simulink model "CC_sfun"  (R2024b)
settings: Solver=FixedStepDiscrete  StartTime=0.0  StopTime=inf  RelTol=1e-3  EnableMultiTasking=on
undefined symbols (not defined in the file or in its folder): CCOk_stepSize
settings Model: TunableVars=CCOk_stepSize  TunableVarsStorageClass=Auto  Creator=nctzv8  LastModifiedBy=voillat
settings ConfigSet: Description=OpenECU configuration set for code generation under RTW-EC.
settings SolverCC: AlgebraicLoopSolver=TrustRegion  PositivePriorityOrder=on
settings DataIOCC: LimitDataPoints=on  SaveFormat=Array  SignalLoggingSaveFormat=ModelDataLogs
settings OptimizationCC: DefaultParameterBehavior=Inlined  InlineInvariantSignals=on  ExpressionDepthLimit=2147483647  StateBitsets=on  DataBitsets=on  ZeroExternalMemoryAtStartup=off  ZeroInternalMemoryAtStartup=off  NoFixptDivByZeroProtection=on  EfficientFloat2IntCast=on  LifeSpan=1  EfficientTunableParamExpr=on
settings DebuggingCC: SaveWithParameterizedLinksMsg=none  SignalResolutionControl=TryResolveAllWithWarning  MultiTaskDSMMsg=warning  MultiTaskCondExecSysMsg=none  SingleTaskRateTransMsg=error  CheckMatrixSingularityMsg=warning  VectorMatrixConversionMsg=warning  SignalLabelMismatchMsg=warning  UnconnectedInputMsg=warning  UnconnectedOutputMsg=warning  UnconnectedLineMsg=warning  AllowSymbolicDim=off  StateNameClashWarn=warning  SFUnexpectedBacktrackingDiag=warning  SFNoUnconditionalDefaultTransitionDiag=warning  SFExecutionAtInitializationDiag=none  ArithmeticOperatorsInVariantConditions=warning
settings HardwareCC: ProdBitPerPointer=32  ProdBitPerSizeT=32  ProdBitPerPtrDiffT=32  ProdLargestAtomicInteger=Long  ProdLargestAtomicFloat=Double  ProdEndianess=BigEndian  ProdWordSize=32  ProdHWDeviceType=Freescale->32-bit PowerPC  TargetIntDivRoundTo=Zero  TargetEndianess=BigEndian  TargetHWDeviceType=Freescale->32-bit PowerPC  ProdEqTarget=off
settings ModelReferenceCC: EnableRefExpFcnMdlSchedulingChecks=on  PropagateSignalLabelsOutOfModel=off
settings SFSimCC: SimUseLocalCustomCode=off  MATLABDynamicMemAlloc=off  CustomCodeUndefinedFunction=UseInterfaceOnly
settings RTWCC: Description=OpenECU Platform Target (ERT, optimised floating-point code)  SystemTargetFile=openecu_ert.tlc  MakeCommand=make_rtw optimized_floating_point=1  TemplateMakefile=openecu_ert_r2015b_64.tmf  RetainRTWFile=on  RTWUseLocalCustomCode=off  IncludeHyperlinkInReport=on  GPUComputeCapability=3.5
settings CodeAppCC: ForceParamTrailComments=on  IgnoreCustomStorageClasses=off  SimulinkDataObjDesc=on  CustomSymbolStrType=$N$R$M  InsertBlockDesc=on  StateflowObjectComments=on  InternalIdentifier=Classic
settings STFCustomTargetCC: TargetLibSuffix=.a  GenerateSampleERTMain=on  IncludeMdlTerminateFcn=off  CombineOutputUpdateFcns=on  IncludeFileDelimiter=UseQuote  ERTCustomFileBanners=on  SupportContinuousTime=off  RemoveResetFunc=on  MATLABClassNameForMDSCustomization=Simulink.SoftwareTarget.ERTCustomization  SystemTargetFile=openecu_ert.tlc
settings ERTTargetCC: MultiwordLength=2048  GenerateSampleERTMain=on  ParMdlRefBuildCompliant=off  CompOptLevelCompliant=off  ConcurrentExecutionCompliant=off  IncludeMdlTerminateFcn=off  IncludeFileDelimiter=UseQuote  SupportNonInlinedSFcns=on  ModelStepFunctionPrototypeControlCompliant=off  CPPClassGenCompliant=off  UseToolchainInfoCompliant=off  ExtModeMexFile=noextcomm  ERTSrcFileBannerTemplate=oe_code_c_template.cgt  ERTHdrFileBannerTemplate=oe_code_h_template.cgt  ERTDataSrcFileTemplate=oe_data_c_template.cgt  ERTDataHdrFileTemplate=oe_data_h_template.cgt  ERTCustomFileTemplate=example_file_process.tlc  GlobalDataDefinition=InSeparateSourceFile  GlobalDataReference=InSeparateHeaderFile  ConvertIfToSwitch=off  SuppressUnreachableDefaultCases=off  EnableUserReplacementTypes=on  DynamicArrayContainerType=coder::array
settings ConfigComp: CovMetricSettings=dw  CovSaveCumulativeToWorkspaceVar=on  CovSaveSingleToWorkspaceVar=on  CovExternalEMLEnable=off

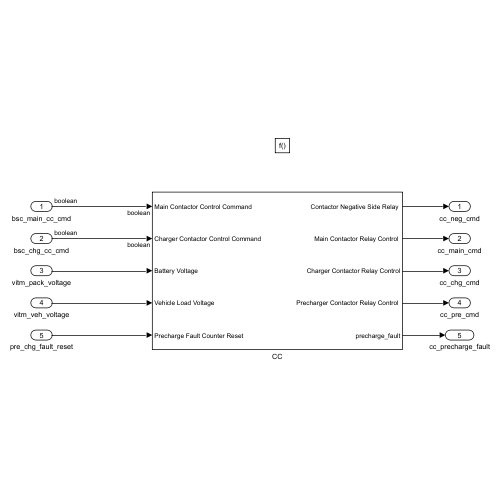
[thumbnail: Simulink's stored preview of the top-level diagram]
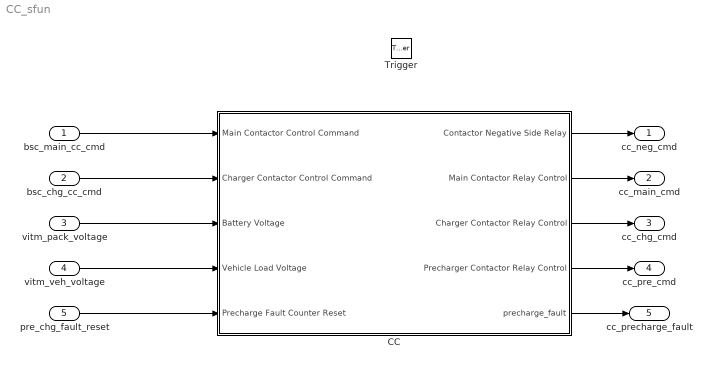
== system CC_sfun ==
  bsc_main_cc_cmd : Inport  OutDataTypeStr=boolean
  bsc_chg_cc_cmd : Inport  Port=2  OutDataTypeStr=boolean
  vitm_pack_voltage : Inport  Port=3
  vitm_veh_voltage : Inport  Port=4
  pre_chg_fault_reset : Inport  Port=5
  Trigger : TriggerPort  TriggerType=function-call  VariantControl=(inherit)  PortDimensions=1
  CC : Subsystem  mask{sfcnParam1=CCOk_stepSize}
      mask prompts: sfcnParam1 "CCOk_stepSize:"
      mask help: Simulink:masks:GenSFuncDesc_MD
      mask Help: eval('feval(''rtwprivate'',''rtwhelpview'',''rtw_sfcn_block'')');
  cc_neg_cmd : Outport
  cc_main_cmd : Outport  Port=2
  cc_chg_cmd : Outport  Port=3
  cc_pre_cmd : Outport  Port=4
  cc_precharge_fault : Outport  Port=5
  wires:
  bsc_main_cc_cmd/1 -> CC/1(Main Contactor Control Command)
  bsc_chg_cc_cmd/1 -> CC/2(Charger Contactor Control Command)
  vitm_pack_voltage/1 -> CC/3(Battery Voltage)
  vitm_veh_voltage/1 -> CC/4(Vehicle Load Voltage)
  pre_chg_fault_reset/1 -> CC/5(Precharge Fault Counter Reset)
  CC/1("Contactor Negative Side Relay ") -> cc_neg_cmd/1
  CC/2("Main Contactor Relay Control ") -> cc_main_cmd/1
  CC/3(Charger Contactor Relay Control) -> cc_chg_cmd/1
  CC/4("Precharger Contactor Relay Control ") -> cc_pre_cmd/1
  CC/5(precharge_fault) -> cc_precharge_fault/1

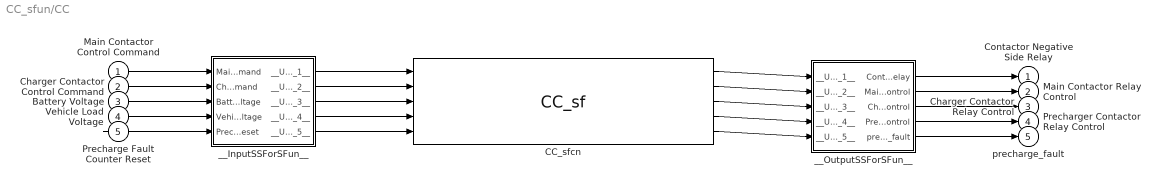
== system CC_sfun/CC ==
  Main Contactor Control Command : Inport  OutDataTypeStr=boolean
  Charger Contactor Control Command : Inport  Port=2  OutDataTypeStr=boolean
  Battery Voltage : Inport  Port=3
  Vehicle Load Voltage : Inport  Port=4
  Precharge Fault Counter Reset : Inport  Port=5
  CC_sfcn : S-Function  FunctionName=CC_sf  Parameters=sfcnParam1  SFunctionModules=""  SFunctionDeploymentMode=off  EnableBusSupport=off  mask{rtw_sf_name=CC_sf, showVar=off, sfcnParam1=sfcnParam1}
      mask prompts: rtw_sf_name "Simulink:masks:GenSFuncName_MP"; showVar "Simulink:masks:GenSFuncShowModuleList_MP"; sfcnParam1 "CCOk_stepSize:"
      mask help: Simulink:masks:GenSFuncDesc_MD
      mask init:
      | displist = '';
      | if ~strcmp(get_param(gcb, 'FunctionName'), rtw_sf_name);
      |   set_param(gcb, 'FunctionName', rtw_sf_name);
      | end
      | % Check if we are generating code
      | rtw_mode = false;
      | if strcmpi(get_param(bdroot(gcb),'SimulationStatus'),'Initializing')
      | 	rtw_mode = strcmpi(get_param(bdroot(gcb),'BuildingRTWCode'),'on') && ...
      | 		~strcmpi(get_param(bdroot(gcb),'TargetStyle'),'SimulationTarget');
      | end
      | if showVar || rtw_mode
      | 	if exist('rtwsfunc') == 2 | exist('rtwsfunc') == 6
      | 		tmplist = rtwsfunc(rtw_sf_name,gcb);
      | 		tmplist = DAStudio.message('Simulink:masks:GenSFuncListOfModules_IC', tmplist);
      | 	elseif showVar
      | 		tmplist1 = DAStudio.message('Simulink:masks:GenSFuncListOfModules_IC', '');
      |         tmplist2 = DAStudio.message('Simulink:masks:GenSFuncNotLicensed_IC');
      |         tmplist = [tmplist1 tmplist2];
      |  	end
      | end
      | if showVar
      |   displist = tmplist;
      | end
      settings: CopyFcn=|
      | if ~strcmp(get_param(gcb,'Linkstatus'),'none') && ...
      | ~strcmp(get_param(gcb,'Linkstatus'),'implicit')
      |   set_param(gcb,'LinkStatus','none');
      | end
      mask Help: eval('feval(''rtwprivate'',''rtwhelpview'',''rtw_sfcn_block'')');
      mask Display:
      | port_label('input',1,'Main Contactor Control Command');
      | port_label('input',2,'Charger Contactor Control Command');
      | port_label('input',3,'Battery Voltage');
      | port_label('input',4,'Vehicle Load Voltage');
      | port_label('input',5,'Precharge Fault Counter Reset');
      | port_label('output',1,'Contactor Negative Side Relay ');
      | port_label('output',2,'Main Contactor Relay Control ');
      | port_label('output',3,'Charger Contactor Relay Control');
      | port_label('output',4,'Precharger Contactor Relay Control ');
      | port_label('output',5,'precharge_fault');
  __InputSSForSFun__ : Subsystem
  __OutputSSForSFun__ : Subsystem
  "Contactor Negative Side Relay " : Outport
  "Main Contactor Relay Control " : Outport  Port=2
  Charger Contactor Relay Control : Outport  Port=3
  "Precharger Contactor Relay Control " : Outport  Port=4
  precharge_fault : Outport  Port=5
  wires:
  Main Contactor Control Command/1 -> __InputSSForSFun__/1(Main Contactor Control Command)
  Charger Contactor Control Command/1 -> __InputSSForSFun__/2(Charger Contactor Control Command)
  Battery Voltage/1 -> __InputSSForSFun__/3(Battery Voltage)
  Vehicle Load Voltage/1 -> __InputSSForSFun__/4(Vehicle Load Voltage)
  Precharge Fault Counter Reset/1 -> __InputSSForSFun__/5(Precharge Fault Counter Reset)
  __InputSSForSFun__/1(__UniqueOutportName__1__) -> CC_sfcn/1
  __InputSSForSFun__/2(__UniqueOutportName__2__) -> CC_sfcn/2
  __InputSSForSFun__/3(__UniqueOutportName__3__) -> CC_sfcn/3
  __InputSSForSFun__/4(__UniqueOutportName__4__) -> CC_sfcn/4
  __InputSSForSFun__/5(__UniqueOutportName__5__) -> CC_sfcn/5
  CC_sfcn/1 -> __OutputSSForSFun__/1(__UniqueInportName__1__)
  CC_sfcn/2 -> __OutputSSForSFun__/2(__UniqueInportName__2__)
  CC_sfcn/3 -> __OutputSSForSFun__/3(__UniqueInportName__3__)
  CC_sfcn/4 -> __OutputSSForSFun__/4(__UniqueInportName__4__)
  CC_sfcn/5 -> __OutputSSForSFun__/5(__UniqueInportName__5__)
  __OutputSSForSFun__/1("Contactor Negative Side Relay ") -> "Contactor Negative Side Relay "/1
  __OutputSSForSFun__/2("Main Contactor Relay Control ") -> "Main Contactor Relay Control "/1
  __OutputSSForSFun__/3(Charger Contactor Relay Control) -> Charger Contactor Relay Control/1
  __OutputSSForSFun__/4("Precharger Contactor Relay Control ") -> "Precharger Contactor Relay Control "/1
  __OutputSSForSFun__/5(precharge_fault) -> precharge_fault/1

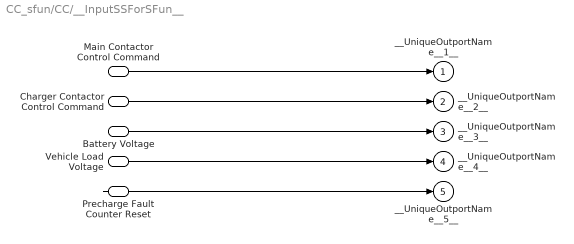
== system CC_sfun/CC/__InputSSForSFun__ ==
  Main Contactor Control Command : Inport  OutDataTypeStr=boolean
  Charger Contactor Control Command : Inport  Port=2  OutDataTypeStr=boolean
  Battery Voltage : Inport  Port=3
  Vehicle Load Voltage : Inport  Port=4
  Precharge Fault Counter Reset : Inport  Port=5
  __UniqueOutportName__1__ : Outport
  __UniqueOutportName__2__ : Outport  Port=2
  __UniqueOutportName__3__ : Outport  Port=3
  __UniqueOutportName__4__ : Outport  Port=4
  __UniqueOutportName__5__ : Outport  Port=5
  wires:
  Main Contactor Control Command/1 -> __UniqueOutportName__1__/1
  Charger Contactor Control Command/1 -> __UniqueOutportName__2__/1
  Battery Voltage/1 -> __UniqueOutportName__3__/1
  Vehicle Load Voltage/1 -> __UniqueOutportName__4__/1
  Precharge Fault Counter Reset/1 -> __UniqueOutportName__5__/1

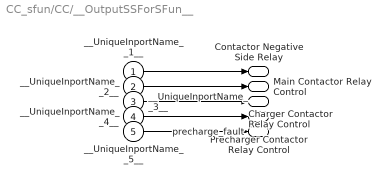
== system CC_sfun/CC/__OutputSSForSFun__ ==
  __UniqueInportName__1__ : Inport
  __UniqueInportName__2__ : Inport  Port=2
  __UniqueInportName__3__ : Inport  Port=3
  __UniqueInportName__4__ : Inport  Port=4
  __UniqueInportName__5__ : Inport  Port=5
  "Contactor Negative Side Relay " : Outport
  "Main Contactor Relay Control " : Outport  Port=2
  Charger Contactor Relay Control : Outport  Port=3
  "Precharger Contactor Relay Control " : Outport  Port=4
  precharge_fault : Outport  Port=5
  wires:
  __UniqueInportName__1__/1 -> "Contactor Negative Side Relay "/1
  __UniqueInportName__2__/1 -> "Main Contactor Relay Control "/1
  __UniqueInportName__3__/1 -> Charger Contactor Relay Control/1
  __UniqueInportName__4__/1 -> "Precharger Contactor Relay Control "/1
  __UniqueInportName__5__/1 -> precharge_fault/1
